simulink model "surge_controller"  (R2021b)
settings: Solver=VariableStepAuto  StartTime=0.0  StopTime=10.0  RelTol=1e-3
undefined symbols (not defined in the file): surge_d1, surge_d2, surge_lambda, surge_m
settings Model: Creator=simengangstad  LastModifiedBy=simengangstad

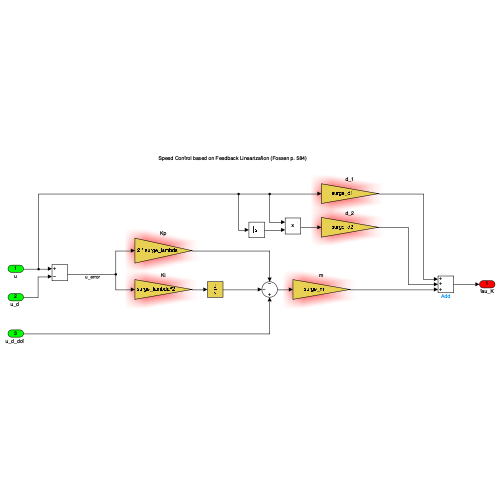
[thumbnail: Simulink's stored preview of the top-level diagram]
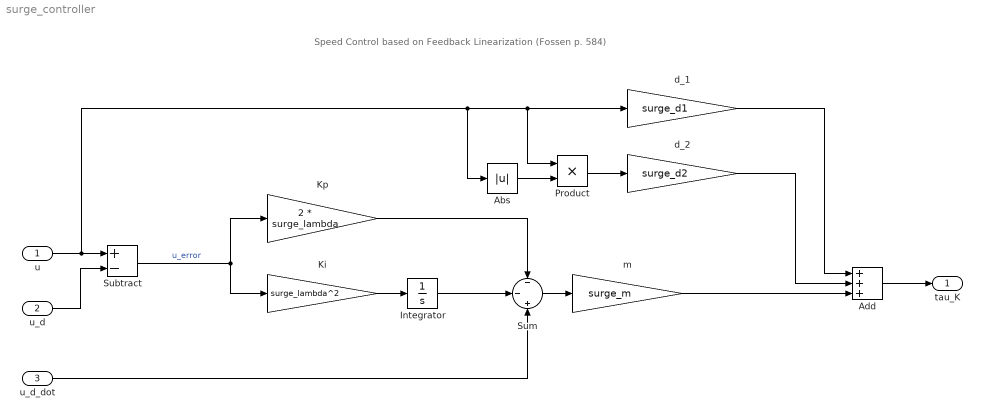
== system surge_controller ==
  note: Speed Control based on Feedback Linearization (Fossen p. 584)
  u : Inport
  "u_d " : Inport  Port=2
  "u_d_dot " : Inport  Port=3
  Abs : Abs
  Add : Sum  Inputs=+++
  Integrator : Integrator
  Ki : Gain  Gain=surge_lambda^2  SaturateOnIntegerOverflow=on  OutDataTypeStr=Inherit: Same as input  ParamDataTypeStr=Inherit: Same as input
  Kp : Gain  Gain=2 * surge_lambda  SaturateOnIntegerOverflow=on  OutDataTypeStr=Inherit: Same as input  ParamDataTypeStr=Inherit: Same as input
  Product : Product
  Subtract : Sum  Inputs=+-
  Sum : Sum  Inputs=-|-|+
  d_1 : Gain  Gain=surge_d1  SaturateOnIntegerOverflow=on  OutDataTypeStr=Inherit: Same as input  ParamDataTypeStr=Inherit: Same as input
  d_2 : Gain  Gain=surge_d2  SaturateOnIntegerOverflow=on  OutDataTypeStr=Inherit: Same as input  ParamDataTypeStr=Inherit: Same as input
  m : Gain  Gain=surge_m  SaturateOnIntegerOverflow=on  OutDataTypeStr=Inherit: Same as input  ParamDataTypeStr=Inherit: Same as input
  tau_K : Outport
  wires:
  Ki/1 -> Integrator/1
  Subtract/1 -> Ki/1, Kp/1  "u_error"
  u/1 -> Abs/1, Product/1, d_1/1, Subtract/1
  "u_d "/1 -> Subtract/2
  "u_d_dot "/1 -> Sum/3
  Integrator/1 -> Sum/2
  Kp/1 -> Sum/1
  Sum/1 -> m/1
  m/1 -> Add/3
  d_2/1 -> Add/2
  d_1/1 -> Add/1
  Abs/1 -> Product/2
  Product/1 -> d_2/1
  Add/1 -> tau_K/1
